simulink model "ham_e"  (R2016a)
settings: Solver=VariableStepAuto  StartTime=0.0  StopTime=10.0  RelTol=1e-3
settings Model: Creator=vuduc  LastModifiedBy=vuduc

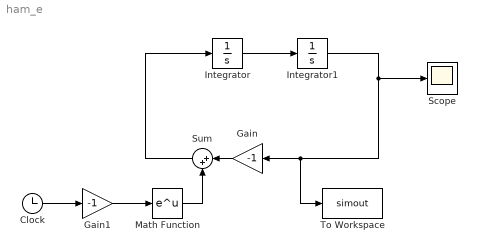
== system ham_e ==
  Clock : Clock
  Gain : Gain  Gain=-1
  Gain1 : Gain  Gain=-1
  Integrator : Integrator  InitialCondition=1
  Integrator1 : Integrator
  Math Function : Math  SaturateOnIntegerOverflow=on
  Scope : Scope
  Sum : Sum  Inputs=|++
  To Workspace : ToWorkspace  VariableName=simout  SaveFormat=Timeseries  SampleTime=-1
  wires:
  Integrator1/1 -> Scope/1, To Workspace/1, Gain/1
  Integrator/1 -> Integrator1/1
  Clock/1 -> Gain1/1
  Gain/1 -> Sum/1
  Math Function/1 -> Sum/2
  Sum/1 -> Integrator/1
  Gain1/1 -> Math Function/1
